simulink model "vechileSimulation"  (R2018a)
settings: Solver=VariableStepAuto  StartTime=0.0  StopTime=10.0  RelTol=1e-3
libraries: fuzblock x1
settings Model: Creator=USER  LastModifiedBy=USER

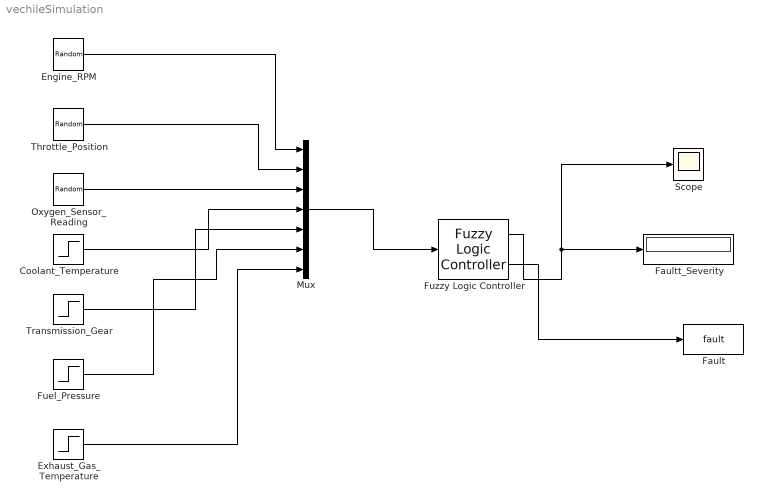
== system vechileSimulation ==
  " Engine_RPM " : UniformRandomNumber  Minimum=1000  Maximum=7000  SampleTime=0.1
  " Fuel_Pressure" : Step  Time=3  Before=15  After=75  SampleTime=0.10  VectorParams1D=off
  " Oxygen_Sensor_Reading " : UniformRandomNumber  Minimum=0.4  Maximum=0.9  SampleTime=0.1
  " Transmission_Gear" : Step  Time=1.5  Before=1  After=4  SampleTime=0.10
  Coolant_Temperature : Step  Time=4  Before=10  After=70  SampleTime=0.9
  Exhaust_Gas_Temperature : Step  Time=3  Before=290  After=880  SampleTime=0.10
  "Fault " : ToWorkspace  VariableName=fault  SaveFormat=Timeseries  SampleTime=-1
  "Faultt_Severity " : Display
  Fuzzy Logic Controller : fuzblock/Fuzzy Logic  Controller  FIS="\"EnginePowertrain\""  OutputSampleNumber=101  DataType=double  FuzzifiedInputs=on  RuleFiringStrengths=off  RuleOutputs=off  AggregatedOutputs=off  SimulateUsing=Interpreted execution  OutOfRangeInputValueMessage=warning  NoRuleFiredMessage=warning  EmptyOutputFuzzySetMessage=warning
  Mux : Mux  Inputs=7
  Scope : Scope
  Throttle_Position : UniformRandomNumber  Minimum=10  Maximum=59  SampleTime=0.1
  wires:
  Coolant_Temperature/1 -> Mux/4
  " Transmission_Gear"/1 -> Mux/5
  " Fuel_Pressure"/1 -> Mux/6
  Exhaust_Gas_Temperature/1 -> Mux/7
  Mux/1 -> Fuzzy Logic Controller/1
  Fuzzy Logic Controller/1 -> Scope/1, "Faultt_Severity "/1
  Fuzzy Logic Controller/2 -> "Fault "/1
  " Engine_RPM "/1 -> Mux/1
  Throttle_Position/1 -> Mux/2
  " Oxygen_Sensor_Reading "/1 -> Mux/3
